simulink model "Airframe_Model_Exercise"  (R2023b)
settings: Solver=VariableStepAuto  StartTime=0.0  StopTime=10  FixedStep=0.002  RelTol=1e-3  EnableMultiTasking=on
libraries: shared6dof x1, robotcorelib x1, uavutilslib x1
settings Model: ExtModeTrigDuration=10000  Creator=plad  LastModifiedBy=plad
settings SolverCC: AlgebraicLoopSolver=TrustRegion  PositivePriorityOrder=on
settings DataIOCC: ReturnWorkspaceOutputs=off
settings OptimizationCC: LifeSpan=inf
settings DebuggingCC: UnconnectedInputMsg=warning  UnconnectedOutputMsg=warning  UnconnectedLineMsg=warning  ArithmeticOperatorsInVariantConditions=warning
settings ModelReferenceCC: EnableRefExpFcnMdlSchedulingChecks=on
settings SFSimCC: SimUseLocalCustomCode=off  CustomCodeUndefinedFunction=UseInterfaceOnly
settings RTWCC: Description=QUARC Win64 Target  SystemTargetFile=quarc_win64.tlc  TemplateMakefile=quarc_default_tmf  RTWUseLocalCustomCode=off
settings CodeAppCC: StateflowObjectComments=on
settings STFCustomTargetCC: TargetPreCompLibLocation=C:\PROGRA~3\QUARC\lib\2016a\win64\release  ConcurrentExecutionCompliant=on  GRTInterface=on  SystemTargetFile=quarc_win64.tlc
settings GRTTargetCC: TargetPreCompLibLocation=C:\PROGRA~3\QUARC\lib\2016a\win64\release  ParMdlRefBuildCompliant=off  CompOptLevelCompliant=off  CombineOutputUpdateFcns=off  MatFileLogging=off  CPPClassGenCompliant=off  GRTInterface=on  UseToolchainInfoCompliant=off  ExtMode=on  ExtModeMexFile=quarc_comm
settings ConfigComp: CovMetricSettings=dswe

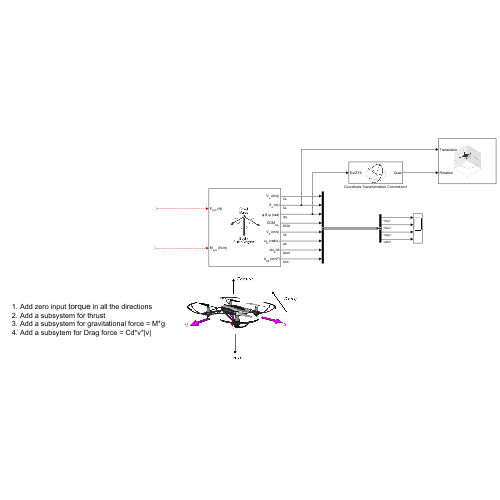
[thumbnail: Simulink's stored preview of the top-level diagram]
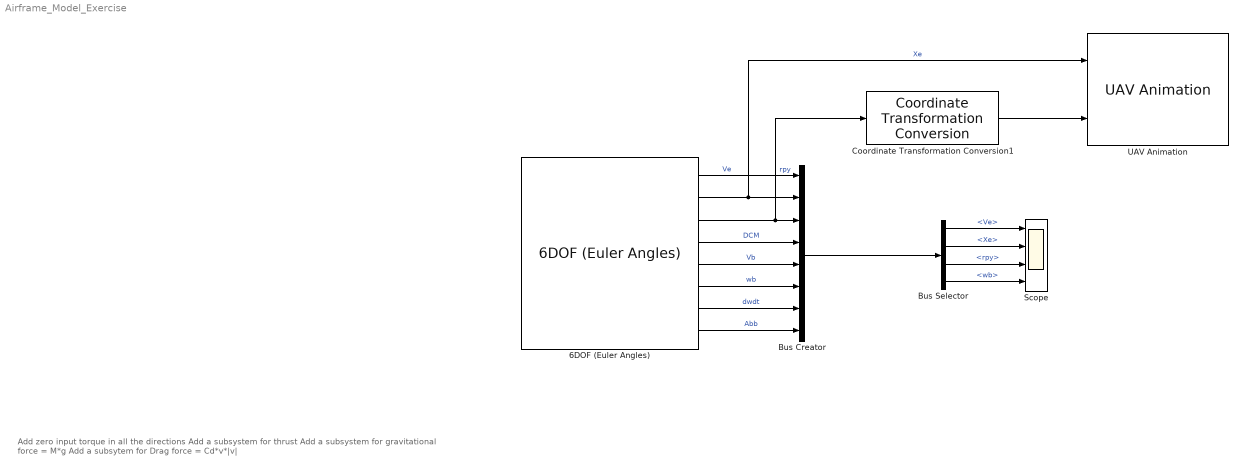
== system Airframe_Model_Exercise ==
  note: Add zero input torque in all the directions
      | Add a subsystem for thrust
      | Add a subsystem for gravitational force = M*g
      | Add a subsytem for Drag force = Cd*v*|v|
  6DOF (Euler Angles) : shared6dof/6DOF (Euler Angles)  units=Metric (MKS)  mtype=Fixed  rep=Euler Angles  xme_0=[0 0 0]  Vm_0=[0 0 0]  eul_0=[0 0 0]  pm_0=[0 0 0]  mass_0=1.0  mass_e=0.5  mass_f=2.0  inertia=eye(3)  inertia_e=eye(3)  inertia_f=2*eye(3)  k_quat=1.0  vre_flag=on  abi_flag=off  aMode=0  xme_statename=''  Vm_statename=''  eul_statename=''  quat_statename=''  pm_statename=''  mass_statename=''
  Bus Creator : BusCreator  Inputs=8
  Bus Selector : BusSelector  OutputSignals=Ve,Xe,rpy,wb
  Coordinate Transformation Conversion1 : robotcorelib/Coordinate Transformation Conversion  InputRepresentation=Euler Angles  InputEulerSequence=ZYX  ShowTrVecInputPort=on  OutputRepresentation=Quaternion  OutputEulerSequence=ZYX  ShowTrVecOutputPort=on  SimulateUsing=Interpreted execution
      settings: LibrarySourceBlock=uavutilslib/Coordinate Transformation Conversion
  Scope : Scope  NumInputPorts=4
  UAV Animation : uavutilslib/UAV Animation  UAVType=Multirotor  UAVSize=1  InertialZDirection=Down  SampleTime=-1
  wires:
  Bus Selector/3 -> Scope/3  "<rpy>"
  6DOF (Euler Angles)/5 -> Bus Creator/5  "Vb"
  Bus Selector/1 -> Scope/1  "<Ve>"
  Bus Creator/1 -> Bus Selector/1
  Bus Selector/4 -> Scope/4  "<wb>"
  6DOF (Euler Angles)/8 -> Bus Creator/8  "Abb"
  6DOF (Euler Angles)/1 -> Bus Creator/1  "Ve"
  6DOF (Euler Angles)/4 -> Bus Creator/4  "DCM"
  6DOF (Euler Angles)/6 -> Bus Creator/6  "wb"
  6DOF (Euler Angles)/2 -> UAV Animation/1, Bus Creator/2  "Xe"
  6DOF (Euler Angles)/3 -> Coordinate Transformation Conversion1/1, Bus Creator/3  "rpy"
  6DOF (Euler Angles)/7 -> Bus Creator/7  "dwdt"
  Bus Selector/2 -> Scope/2  "<Xe>"
  Coordinate Transformation Conversion1/1 -> UAV Animation/2
  ? -> 6DOF (Euler Angles)/1
  ? -> 6DOF (Euler Angles)/2
